simulink model "task9_lab14"  (R2021a)
settings: Solver=VariableStepAuto  StartTime=0.0  StopTime=10.0  RelTol=1e-3
settings Model: Creator=reemb  LastModifiedBy=reemb

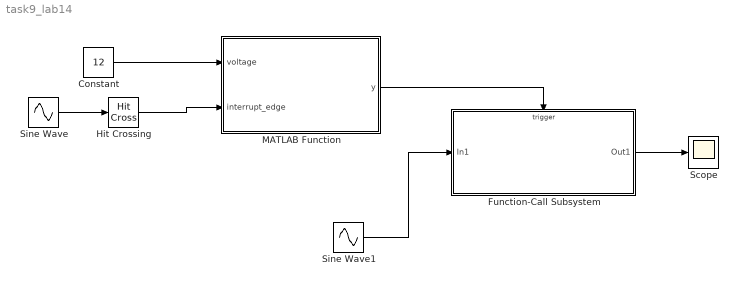
== system task9_lab14 ==
  Constant : Constant  Value=12
  Function-Call Subsystem : Subsystem  TreatAsAtomicUnit=on
  Hit Crossing : HitCross
  MATLAB Function : MATLAB Function  TreatAsAtomicUnit=on
  Scope : Scope
  Sine Wave : Sin  SampleTime=0
  Sine Wave1 : Sin  SampleTime=0
  wires:
  Function-Call Subsystem/1(Out1) -> Scope/1
  Sine Wave/1 -> Hit Crossing/1
  MATLAB Function/1(y) -> Function-Call Subsystem/Trigger
  Hit Crossing/1 -> MATLAB Function/2(interrupt_edge)
  Sine Wave1/1 -> Function-Call Subsystem/1(In1)
  Constant/1 -> MATLAB Function/1(voltage)

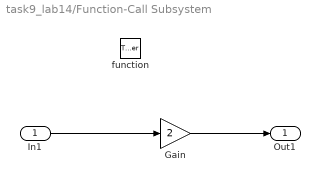
== system task9_lab14/Function-Call Subsystem ==
  In1 : Inport
  function : TriggerPort  TriggerType=function-call  VariantControl=(inherit)
  Gain : Gain  Gain=2
  Out1 : Outport
  wires:
  Gain/1 -> Out1/1
  In1/1 -> Gain/1

== matlab function task9_lab14/MATLAB Function ==
  data: voltage input; y output; interrupt_edge input
function y = fcn( voltage, interrupt_edge)


y = false; 

if (voltage > 10) && (interrupt_edge == 1)
    y = true; 
end
